simulink model "PulseNeuronMembraneCapacityTest"  (Simulink 7.5)
settings: Solver=ode45  StartTime=0.0  StopTime=10  RelTol=1e-3
libraries: NeuroModelerLibrary x12, simulink x1
settings Model: Creator=Bakhshiev  LastModifiedBy=Bakhshiev

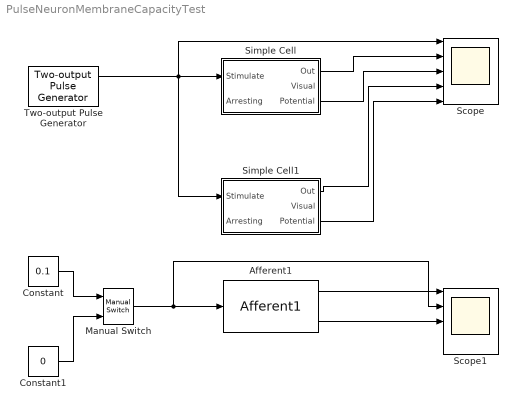
== system PulseNeuronMembraneCapacityTest ==
  Afferent1 : NeuroModelerLibrary/Simple Cells/Afferent1  SystemSampleTime=-1
  Constant : Constant  Value=0.1  OutDataType=fixdt(1, 16)  OutScaling=2^0
  Constant1 : Constant  Value=0  OutDataType=fixdt(1, 16)  OutScaling=2^0
  Manual Switch : simulink/Signal Routing/Manual Switch  SystemSampleTime=-1  sw=0  action=0  varsize=off
  Scope : Scope  NumInputPorts=5
      settings: YMin=-1~-1~-1~-1~0  YMax=1~1~1~1~3e-005  MaxDataPoints=500000
  Scope1 : Scope  NumInputPorts=5
      settings: YMin=-1~-1~-1~-1~-1  YMax=1~1~0~1~1  SaveName=ScopeData2  MaxDataPoints=500000
  Simple Cell : Subsystem  AncestorBlock=NeuroModelerLibrary/Simple Cells/Simple Cell
  Simple Cell1 : Subsystem  AncestorBlock=NeuroModelerLibrary/Simple Cells/Simple Cell
  Two-output Pulse Generator : NeuroModelerLibrary/Support/Two-output Pulse Generator  SystemSampleTime=-1  A=1  P1=300  P2=200  PW=1  ST=0.001  OOn1=5  OOff1=7  OOn2=1.1  OOff2=1.2
  wires:
  Two-output Pulse Generator/1 -> Simple Cell/1(Stimulate), Scope/1, Simple Cell1/1(Stimulate)
  Simple Cell/1(Out) -> Scope/2
  Simple Cell1/3(Potential) -> Scope/5
  Simple Cell/3(Potential) -> Scope/3
  Simple Cell1/1(Out) -> Scope/4
  Afferent1/1 -> Scope1/1
  Afferent1/3 -> Scope1/3
  Constant1/1 -> Manual Switch/2
  Constant/1 -> Manual Switch/1
  Manual Switch/1 -> Afferent1/1, Scope1/2

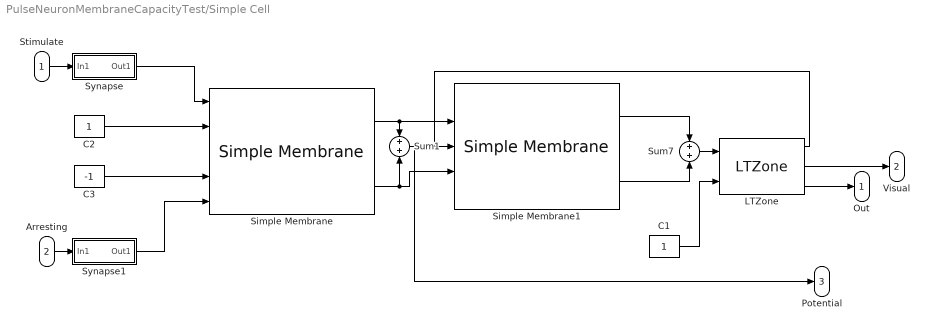
== system PulseNeuronMembraneCapacityTest/Simple Cell ==
  Stimulate : Inport  OutDataType=sfix(16)  OutScaling=2^0
  Arresting : Inport  Port=2  OutDataType=sfix(16)  OutScaling=2^0
  C1 : Constant  OutDataType=sfix(16)  OutScaling=2^0
  C2 : Constant  OutDataType=sfix(16)  OutScaling=2^0
  C3 : Constant  Value=-1  OutDataType=sfix(16)  OutScaling=2^0
  LTZone : NeuroModelerLibrary/Neuron Elements/LTZone  SystemSampleTime=-1  NM=1  FB=1.7  IT=0.005  T=0.00001
  Simple Membrane : NeuroModelerLibrary/Neuron Elements/Simple Membrane  SystemSampleTime=-1  ACm=1e-9  ARm=1e7  ECm=1e-9  ERm=1e7  ARFm=1e8  ERFm=1e8
  Simple Membrane1 : NeuroModelerLibrary/Neuron Elements/Simple Membrane  SystemSampleTime=-1  ACm=1e-7  ARm=1e7  ECm=1e-7  ERm=1e7  ARFm=1e8  ERFm=1e8
  Sum1 : Sum  OutDataType=sfix(16)  OutScaling=2^0  SaturateOnIntegerOverflow=on  InputSameDT=on  OutDataTypeStr=Inherit: Same as first input
  Sum7 : Sum  OutDataType=sfix(16)  OutScaling=2^0  SaturateOnIntegerOverflow=on  InputSameDT=on  OutDataTypeStr=Inherit: Same as first input
  Synapse : Subsystem  AncestorBlock=NeuroModelerLibrary/Neuron Elements/Synapse  mask{SecretionTC=0.001, DecompositionTC=0.01, ksi=2, gamma=1e8}
      mask prompts: SecretionTC "Mediator Secretion"; DecompositionTC "Mediator Decomposition"
  Synapse1 : Subsystem  AncestorBlock=NeuroModelerLibrary/Neuron Elements/Synapse  mask{SecretionTC=0.001, DecompositionTC=0.01, ksi=2, gamma=1e8}
      mask prompts: SecretionTC "Mediator Secretion"; DecompositionTC "Mediator Decomposition"
  Out : Outport  OutDataType=sfix(16)  OutScaling=2^0
  Visual : Outport  Port=2  OutDataType=sfix(16)  OutScaling=2^0
  Potential : Outport  Port=3  OutDataType=sfix(16)  OutScaling=2^0
  wires:
  Synapse1/1(Out1) -> Simple Membrane/5
  Synapse/1(Out1) -> Simple Membrane/1
  C3/1 -> Simple Membrane/4
  C2/1 -> Simple Membrane/2
  Sum7/1 -> LTZone/1
  Arresting/1 -> Synapse1/1(In1)
  Stimulate/1 -> Synapse/1(In1)
  C1/1 -> LTZone/2
  LTZone/3 -> Out/1
  LTZone/2 -> Visual/1
  Simple Membrane/1 -> Simple Membrane1/2, Sum1/1
  Simple Membrane/2 -> Simple Membrane1/4, Sum1/2
  Simple Membrane1/1 -> Sum7/1
  Simple Membrane1/2 -> Sum7/2
  LTZone/1 -> Simple Membrane1/3
  Sum1/1 -> Potential/1

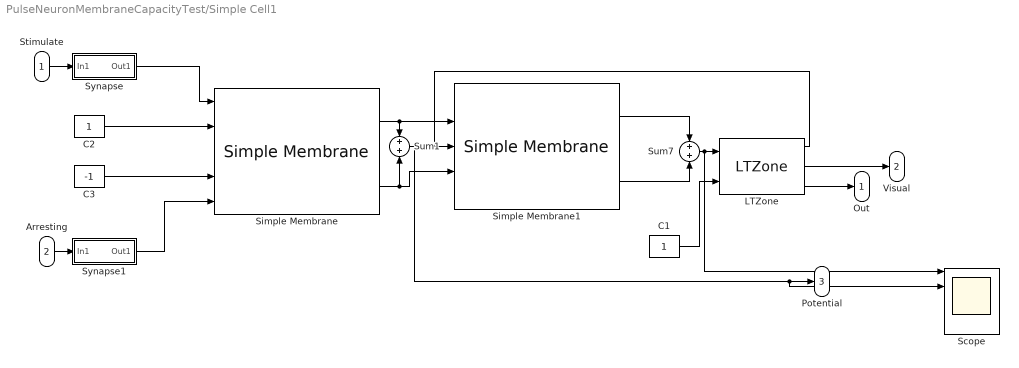
== system PulseNeuronMembraneCapacityTest/Simple Cell1 ==
  Stimulate : Inport  OutDataType=sfix(16)  OutScaling=2^0
  Arresting : Inport  Port=2  OutDataType=sfix(16)  OutScaling=2^0
  C1 : Constant  OutDataType=sfix(16)  OutScaling=2^0
  C2 : Constant  OutDataType=sfix(16)  OutScaling=2^0
  C3 : Constant  Value=-1  OutDataType=sfix(16)  OutScaling=2^0
  LTZone : NeuroModelerLibrary/Neuron Elements/LTZone  SystemSampleTime=-1  NM=1  FB=1.7  IT=0.005  T=0.00001
  Scope : Scope  NumInputPorts=5
      settings: YMin=-0.002~-1~-1~-1~-1  YMax=0.00025~1~1~1~1  MaxDataPoints=500000
  Simple Membrane : NeuroModelerLibrary/Neuron Elements/Simple Membrane  SystemSampleTime=-1  ACm=1e-7  ARm=1e7  ECm=1e-7  ERm=1e7  ARFm=1e8  ERFm=1e8
  Simple Membrane1 : NeuroModelerLibrary/Neuron Elements/Simple Membrane  SystemSampleTime=-1  ACm=1e-7  ARm=1e7  ECm=1e-7  ERm=1e7  ARFm=1e8  ERFm=1e8
  Sum1 : Sum  OutDataType=sfix(16)  OutScaling=2^0  SaturateOnIntegerOverflow=on  InputSameDT=on  OutDataTypeStr=Inherit: Same as first input
  Sum7 : Sum  OutDataType=sfix(16)  OutScaling=2^0  SaturateOnIntegerOverflow=on  InputSameDT=on  OutDataTypeStr=Inherit: Same as first input
  Synapse : Subsystem  AncestorBlock=NeuroModelerLibrary/Neuron Elements/Synapse  mask{SecretionTC=0.001, DecompositionTC=0.01, ksi=2, gamma=1e8}
      mask prompts: SecretionTC "Mediator Secretion"; DecompositionTC "Mediator Decomposition"
  Synapse1 : Subsystem  AncestorBlock=NeuroModelerLibrary/Neuron Elements/Synapse  mask{SecretionTC=0.001, DecompositionTC=0.01, ksi=2, gamma=1e8}
      mask prompts: SecretionTC "Mediator Secretion"; DecompositionTC "Mediator Decomposition"
  Out : Outport  OutDataType=sfix(16)  OutScaling=2^0
  Visual : Outport  Port=2  OutDataType=sfix(16)  OutScaling=2^0
  Potential : Outport  Port=3  OutDataType=sfix(16)  OutScaling=2^0
  wires:
  Synapse1/1(Out1) -> Simple Membrane/5
  Synapse/1(Out1) -> Simple Membrane/1
  C3/1 -> Simple Membrane/4
  C2/1 -> Simple Membrane/2
  Sum7/1 -> LTZone/1, Scope/1
  Arresting/1 -> Synapse1/1(In1)
  Stimulate/1 -> Synapse/1(In1)
  C1/1 -> LTZone/2
  LTZone/3 -> Out/1
  LTZone/2 -> Visual/1
  Simple Membrane/1 -> Simple Membrane1/2, Sum1/1
  Simple Membrane/2 -> Simple Membrane1/4, Sum1/2
  Simple Membrane1/1 -> Sum7/1
  Simple Membrane1/2 -> Sum7/2
  LTZone/1 -> Simple Membrane1/3
  Sum1/1 -> Potential/1, Scope/2

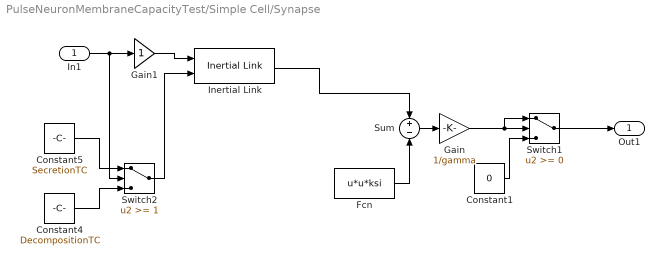
== system PulseNeuronMembraneCapacityTest/Simple Cell/Synapse ==
  In1 : Inport  OutDataType=sfix(16)  OutScaling=2^0
  Constant1 : Constant  Value=0  OutDataType=sfix(16)  OutScaling=2^0
  Constant4 : Constant  Value=DecompositionTC  OutDataType=sfix(16)  OutScaling=2^0
  Constant5 : Constant  Value=SecretionTC  OutDataType=sfix(16)  OutScaling=2^0
  Fcn : Fcn  Expr=u*u*ksi
  Gain : Gain  Gain=1/gamma  ParameterDataType=sfix(16)  ParameterScaling=2^0  OutDataType=sfix(16)  OutScaling=2^0  SaturateOnIntegerOverflow=on  OutDataTypeStr=Inherit: Same as input  ParamDataTypeStr=Inherit: Same as input
  Gain1 : Gain  ParameterDataType=sfix(16)  ParameterScaling=2^0  OutDataType=sfix(16)  OutScaling=2^0  SaturateOnIntegerOverflow=on  OutDataTypeStr=Inherit: Same as input  ParamDataTypeStr=Inherit: Same as input
  Inertial Link : NeuroModelerLibrary/Support/Inertial Link  SystemSampleTime=-1
  Sum : Sum  Inputs=+-  OutDataType=sfix(16)  OutScaling=2^0  SaturateOnIntegerOverflow=on
  Switch1 : Switch
  Switch2 : Switch  Threshold=1
  Out1 : Outport  OutDataType=sfix(16)  OutScaling=2^0
  wires:
  Switch1/1 -> Out1/1
  Gain1/1 -> Inertial Link/1
  Constant1/1 -> Switch1/3
  Gain/1 -> Switch1/1, Switch1/2
  Switch2/1 -> Inertial Link/2
  Constant5/1 -> Switch2/1
  Constant4/1 -> Switch2/3
  Inertial Link/1 -> Sum/1
  Sum/1 -> Gain/1
  In1/1 -> Gain1/1, Switch2/2
  Fcn/1 -> Sum/2

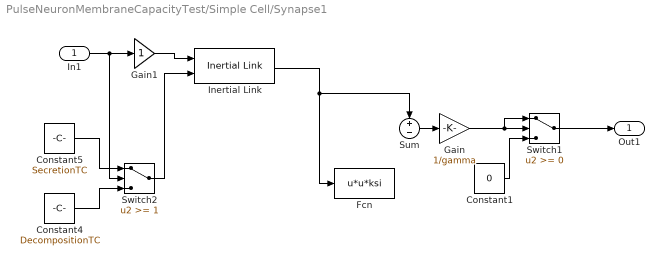
== system PulseNeuronMembraneCapacityTest/Simple Cell/Synapse1 ==
  In1 : Inport  OutDataType=sfix(16)  OutScaling=2^0
  Constant1 : Constant  Value=0  OutDataType=sfix(16)  OutScaling=2^0
  Constant4 : Constant  Value=DecompositionTC  OutDataType=sfix(16)  OutScaling=2^0
  Constant5 : Constant  Value=SecretionTC  OutDataType=sfix(16)  OutScaling=2^0
  Fcn : Fcn  Expr=u*u*ksi
  Gain : Gain  Gain=1/gamma  ParameterDataType=sfix(16)  ParameterScaling=2^0  OutDataType=sfix(16)  OutScaling=2^0  SaturateOnIntegerOverflow=on  OutDataTypeStr=Inherit: Same as input  ParamDataTypeStr=Inherit: Same as input
  Gain1 : Gain  ParameterDataType=sfix(16)  ParameterScaling=2^0  OutDataType=sfix(16)  OutScaling=2^0  SaturateOnIntegerOverflow=on  OutDataTypeStr=Inherit: Same as input  ParamDataTypeStr=Inherit: Same as input
  Inertial Link : NeuroModelerLibrary/Support/Inertial Link  SystemSampleTime=-1
  Sum : Sum  Inputs=+-  OutDataType=sfix(16)  OutScaling=2^0  SaturateOnIntegerOverflow=on
  Switch1 : Switch
  Switch2 : Switch  Threshold=1
  Out1 : Outport  OutDataType=sfix(16)  OutScaling=2^0
  wires:
  Switch1/1 -> Out1/1
  Gain1/1 -> Inertial Link/1
  Constant1/1 -> Switch1/3
  Gain/1 -> Switch1/1, Switch1/2
  Switch2/1 -> Inertial Link/2
  Constant5/1 -> Switch2/1
  Constant4/1 -> Switch2/3
  Inertial Link/1 -> Sum/1, Fcn/1
  Sum/1 -> Gain/1
  In1/1 -> Gain1/1, Switch2/2

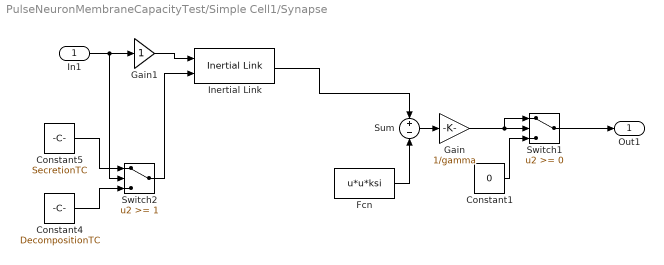
== system PulseNeuronMembraneCapacityTest/Simple Cell1/Synapse ==
  In1 : Inport  OutDataType=sfix(16)  OutScaling=2^0
  Constant1 : Constant  Value=0  OutDataType=sfix(16)  OutScaling=2^0
  Constant4 : Constant  Value=DecompositionTC  OutDataType=sfix(16)  OutScaling=2^0
  Constant5 : Constant  Value=SecretionTC  OutDataType=sfix(16)  OutScaling=2^0
  Fcn : Fcn  Expr=u*u*ksi
  Gain : Gain  Gain=1/gamma  ParameterDataType=sfix(16)  ParameterScaling=2^0  OutDataType=sfix(16)  OutScaling=2^0  SaturateOnIntegerOverflow=on  OutDataTypeStr=Inherit: Same as input  ParamDataTypeStr=Inherit: Same as input
  Gain1 : Gain  ParameterDataType=sfix(16)  ParameterScaling=2^0  OutDataType=sfix(16)  OutScaling=2^0  SaturateOnIntegerOverflow=on  OutDataTypeStr=Inherit: Same as input  ParamDataTypeStr=Inherit: Same as input
  Inertial Link : NeuroModelerLibrary/Support/Inertial Link  SystemSampleTime=-1
  Sum : Sum  Inputs=+-  OutDataType=sfix(16)  OutScaling=2^0  SaturateOnIntegerOverflow=on
  Switch1 : Switch
  Switch2 : Switch  Threshold=1
  Out1 : Outport  OutDataType=sfix(16)  OutScaling=2^0
  wires:
  Switch1/1 -> Out1/1
  Gain1/1 -> Inertial Link/1
  Constant1/1 -> Switch1/3
  Gain/1 -> Switch1/1, Switch1/2
  Switch2/1 -> Inertial Link/2
  Constant5/1 -> Switch2/1
  Constant4/1 -> Switch2/3
  Inertial Link/1 -> Sum/1
  Sum/1 -> Gain/1
  In1/1 -> Gain1/1, Switch2/2
  Fcn/1 -> Sum/2

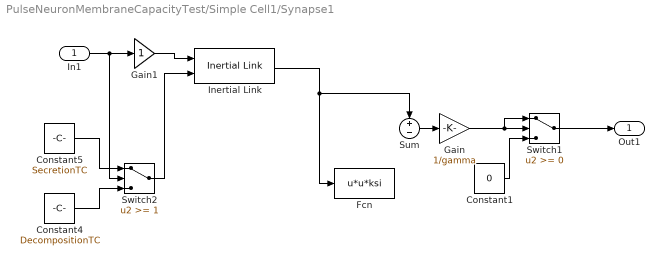
== system PulseNeuronMembraneCapacityTest/Simple Cell1/Synapse1 ==
  In1 : Inport  OutDataType=sfix(16)  OutScaling=2^0
  Constant1 : Constant  Value=0  OutDataType=sfix(16)  OutScaling=2^0
  Constant4 : Constant  Value=DecompositionTC  OutDataType=sfix(16)  OutScaling=2^0
  Constant5 : Constant  Value=SecretionTC  OutDataType=sfix(16)  OutScaling=2^0
  Fcn : Fcn  Expr=u*u*ksi
  Gain : Gain  Gain=1/gamma  ParameterDataType=sfix(16)  ParameterScaling=2^0  OutDataType=sfix(16)  OutScaling=2^0  SaturateOnIntegerOverflow=on  OutDataTypeStr=Inherit: Same as input  ParamDataTypeStr=Inherit: Same as input
  Gain1 : Gain  ParameterDataType=sfix(16)  ParameterScaling=2^0  OutDataType=sfix(16)  OutScaling=2^0  SaturateOnIntegerOverflow=on  OutDataTypeStr=Inherit: Same as input  ParamDataTypeStr=Inherit: Same as input
  Inertial Link : NeuroModelerLibrary/Support/Inertial Link  SystemSampleTime=-1
  Sum : Sum  Inputs=+-  OutDataType=sfix(16)  OutScaling=2^0  SaturateOnIntegerOverflow=on
  Switch1 : Switch
  Switch2 : Switch  Threshold=1
  Out1 : Outport  OutDataType=sfix(16)  OutScaling=2^0
  wires:
  Switch1/1 -> Out1/1
  Gain1/1 -> Inertial Link/1
  Constant1/1 -> Switch1/3
  Gain/1 -> Switch1/1, Switch1/2
  Switch2/1 -> Inertial Link/2
  Constant5/1 -> Switch2/1
  Constant4/1 -> Switch2/3
  Inertial Link/1 -> Sum/1, Fcn/1
  Sum/1 -> Gain/1
  In1/1 -> Gain1/1, Switch2/2
